simulink library "INT_PT_Grip"  (R2016b)
settings: Solver=VariableStepAuto  StartTime=0.0  StopTime=10.0  RelTol=1e-3
settings Model: Creator=Administrator  LastModifiedBy=Administrator

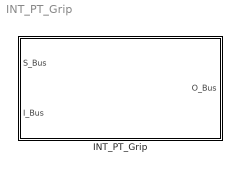
== system INT_PT_Grip ==
  INT_PT_Grip : Subsystem

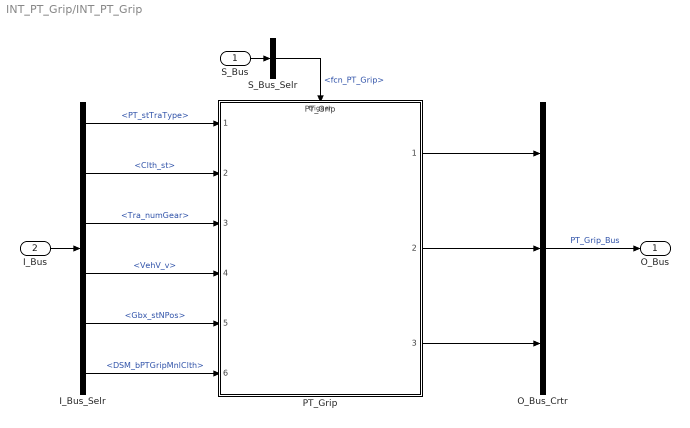
== system INT_PT_Grip/INT_PT_Grip ==
  S_Bus : Inport
  I_Bus : Inport  Port=2
  I_Bus_Selr : BusSelector  OutputSignals=PT_stTraType,Clth_st,Tra_numGear,VehV_v,Gbx_stNPos,DSM_bPTGripMnlClth
  O_Bus_Crtr : BusCreator  Inputs=3
  PT_Grip : ModelReference  ModelNameDialog=PT_Grip  SimulationMode=Normal  ModelReferenceVersion=1.20  TriggerPortName=function  TriggerPortTriggerType=function-call  TriggerPortStatesWhenEnabling=held
  S_Bus_Selr : BusSelector  OutputSignals=fcn_PT_Grip
  O_Bus : Outport
  wires:
  S_Bus_Selr/1 -> PT_Grip/Trigger  "<fcn_PT_Grip>"
  S_Bus/1 -> S_Bus_Selr/1
  I_Bus/1 -> I_Bus_Selr/1
  I_Bus_Selr/1 -> PT_Grip/1  "<PT_stTraType>"
  I_Bus_Selr/2 -> PT_Grip/2  "<Clth_st>"
  I_Bus_Selr/3 -> PT_Grip/3  "<Tra_numGear>"
  I_Bus_Selr/4 -> PT_Grip/4  "<VehV_v>"
  I_Bus_Selr/5 -> PT_Grip/5  "<Gbx_stNPos>"
  I_Bus_Selr/6 -> PT_Grip/6  "<DSM_bPTGripMnlClth>"
  O_Bus_Crtr/1 -> O_Bus/1  "PT_Grip_Bus"
  PT_Grip/1 -> O_Bus_Crtr/1
  PT_Grip/2 -> O_Bus_Crtr/2
  PT_Grip/3 -> O_Bus_Crtr/3
